simulink model "explicitCompFilter_uORB"  (R2024b)
settings: Solver=FixedStepAuto  StartTime=0.0  StopTime=35  FixedStep=0.005  RelTol=1e-3  EnableMultiTasking=on
PreLoadFcn:
  | %b_prev = Simulink.Signal;
  | %q_prev = Simulink.Signal;
  | 
  | %b_prev.InitialValue = '[0; 0; 0]';
  | %q_prev.InitialValue = '[0; 0; 0; 0]';
InitFcn:
  | %g_or = [0;0;-9.81];
  | %m_or = [27.5550; 2.4169; 16.0849];
  | gyroBias = [1; 1; 0.5];
  | 
  | %IF USING BUILT-IN UAV ANIMATION, uncomment below
  | 
  | %CLEAR UAV ANIMATIONS
  | %figHandles = findall(groot, 'Type', 'figure');
  | 
  | %for i=1:size(figHandles)
  | %    figObj = figHandles(i);
  | %    figName = figObj.Name;
  | %   if contains(figName, 'UAV Animation');
  | %        delete(figObj);
  | %    end
  | %end
undefined symbols (not defined in the file): g
libraries: robotcorelib x3, simulink_extras x3, px4Sensorslib x2, simulink x1, matrix_library x1, vrlib x1, px4uORBlib x1
(part 1 of 3)
settings Model: SimulationMode=external  ExtModeTrigDuration=10  Creator=Alyssa  LastModifiedBy=Alyssa
settings SolverCC: PositivePriorityOrder=on
settings OptimizationCC: BlockReduction=off  BooleanDataType=off  EnhancedBackFolding=on  PassReuseOutputArgsAs=Individual arguments  ZeroExternalMemoryAtStartup=off  ZeroInternalMemoryAtStartup=off  MaxStackSize=64  OptimizeBlockOrder=speed  DifferentSizesBufferReuse=on  OptimizationCustomize=off  EfficientTunableParamExpr=on
settings DebuggingCC: SaveWithParameterizedLinksMsg=none  UnderspecifiedInitializationDetection=Classic  MergeDetectMultiDrivingBlocksExec=none  SignalResolutionControl=TryResolveAllWithWarning  ParameterTunabilityLossMsg=error
settings HardwareCC: ProdBitPerPointer=32  ProdBitPerSizeT=32  ProdBitPerPtrDiffT=32  ProdLargestAtomicInteger=Long  ProdLargestAtomicFloat=Double  ProdWordSize=32  ProdLongLongMode=on  ProdHWDeviceType=ARM Compatible->ARM Cortex  TargetLargestAtomicInteger=Long  TargetLargestAtomicFloat=Double  TargetLongLongMode=on  TargetIntDivRoundTo=Zero  TargetEndianess=LittleEndian  TargetHWDeviceType=ARM Compatible->ARM Cortex
settings ModelReferenceCC: PropagateSignalLabelsOutOfModel=off
settings SFSimCC: MATLABDynamicMemAlloc=off  SimTargetLang=C++
settings RTWCC: Description=Embedded Coder  SystemTargetFile=ert.tlc  HardwareBoard=PX4 Pixhawk Series  TLCOptions="-aInlineSetEventsForThisBaseRateFcn=TLC_FALSE -aSuppressMultiTaskScheduler=TLC_FALSE  -aRateBasedStepFcn=0"  TemplateMakefile=ert_default_tmf  Toolchain=GNU Tools for PX4 Autopilots  TargetLang=C++
settings CodeAppCC: ForceParamTrailComments=on  IgnoreCustomStorageClasses=off  OperatorAnnotations=on  SimulinkDataObjDesc=on  SFDataObjDesc=on  InsertBlockDesc=on
settings ERTTargetCC: ExtModeTransport=3  ExtModeStaticAlloc=on  ExtModeStaticAllocSize=1024  ExtModeMexFile=ext_xcp  ExtModeIntrfLevel=Level2 - Open  InlinedParameterPlacement=Hierarchical  RootIOFormat=Structure reference

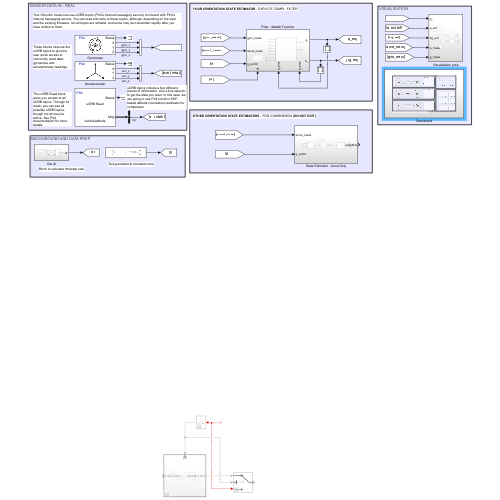
[thumbnail: Simulink's stored preview of the top-level diagram]
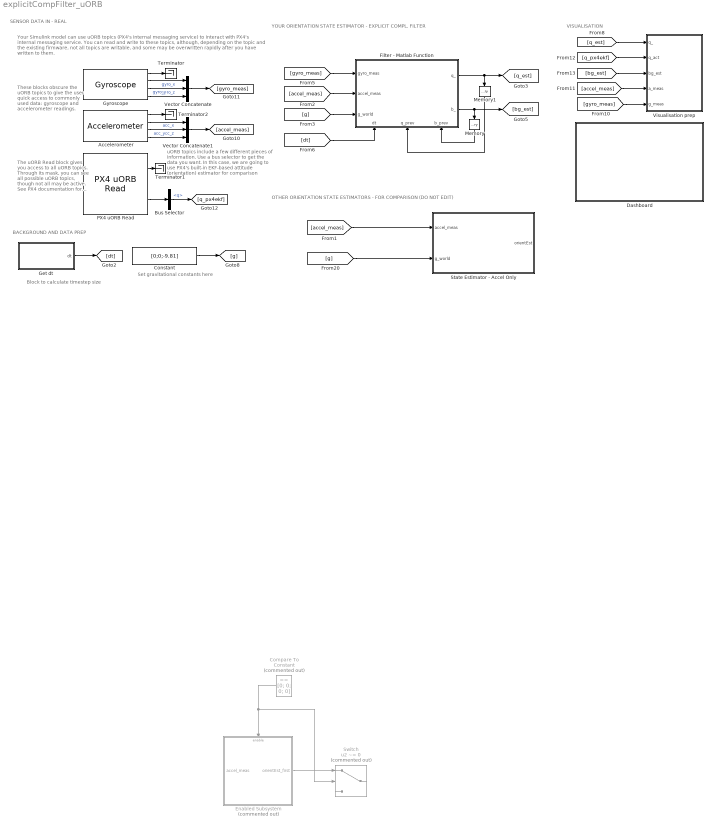
== system explicitCompFilter_uORB ==
  note: Set gravitational constants here
  note: Block to calculate timestep size
  note: uORB topics include a few different pieces of information. Use a bus selector to get the data you want. In this case, we are going to use PX4's built-in EKF-based attitude (orientation) estimator for comparison
  note: Your Simulink model can use uORB topics (PX4's internal messaging service) to interact with PX4's internal messaging service. You can read and write to these topics, although, depending on the topic and the existing firmware, not all topics are writable, and some may be overwritten rapidly after you have written to them.
  note: OTHER ORIENTATION STATE ESTIMATORS - FOR COMPARISON (DO NOT EDIT)
  note: VISUALISATION
  note: YOUR ORIENTATION STATE ESTIMATOR - EXPLICIT COMPL. FILTER
  note: BACKGROUND AND DATA PREP
  note: SENSOR DATA IN - REAL
  note: These blocks obscure the uORB topics to give the user quick access to commonly used data: gyroscope and accelerometer readings.
  note: The uORB Read block gives you access to all uORB topics. Through its mask, you can see all possible uORB topics, though not all may be active. See PX4 documentation for more details.
  Accelerometer : px4Sensorslib/Accelerometer  uorbTimeStamp=off  BlockingMode=off  BlockTimeout=1e-3  sampleTime=0.005
  Bus Selector : BusSelector  OutputSignals=q
  Compare To Constant : simulink/Logic and Bit Operations/Compare To Constant  Commented=on  relop===  const=[0; 0; 0; 0]  OutDataTypeStr=boolean
  Constant : Constant  Value=[0;0;-9.81]
  Dashboard : Subsystem
  Enabled Subsystem : Subsystem  Commented=on  TreatAsAtomicUnit=on
  Filter - Matlab Function : Subsystem
      settings: PortSchema="{\"entries\":[{\"content\":{\"sides\":[{\"content\":{\"connectorIds\":[\"In1\",\"In2\",\"In3\"]},\"type\":\"ConnectorPlacement.EquallySpacedRectSide\",\"uuid\":\"120bcc35-90e2-4731-ad16-59b67db11649\"},{\"content\":{\"connectorIds\":[\"Out1\",\"Out2\"],\"side\":\"RIGHT\"},\"type\":\"ConnectorPlacement.EquallySpacedRectSide\",\"uuid\":\"22d58821-716e-45cf-a51f-08f37bdaf288\"},{\"content\":{\"side\":\"TOP\"},\"type\":\"ConnectorPlacement.EquallySpacedRectSide\",\"uuid\":\"ed81b21f-3f84-420f-a2fc-1eb3e92691bd\"},{\"content\":{\"connectorIds\":[\"In4\",\"In5\",\"In6\"],\"side\":\"BOTTOM\"},\"type\":\"ConnectorPlacement.EquallySpacedRectSide\",\"uuid\":\"91ee1563-cd18-490d-aa8e-820150fc957e\"}]},\"type\":\"ConnectorPlacement.EquallySpacedConnector\",\"uuid\":\"c3e854d1-83c9-4500-85fa-dacad668fd3c\"}],\"packageUris\":[\"http://schema.mathworks.com/mf0/Connector/R2020b\"],\"version\":\"1.0\"}"
  Get dt : Subsystem
  Gyroscope : px4Sensorslib/Gyroscope  uorbTimeStamp=off  BlockingMode=off  BlockTimeout=1e-3  sampleTime=0.005
  Memory : Memory  InitialCondition=[0; 0; 0]
  Memory1 : Memory  InitialCondition=[1; 0; 0; 0]
  PX4 uORB Read : px4uORBlib/PX4 uORB Read  uORBTopic=VehicleAttitude  selectInstance=vehicle_attitude  SampleTime=-1  BlockingMode=off  BlockTimeout=1e-3
  State Estimator - Accel Only : Subsystem
  Switch : Switch  Commented=on  Criteria=u2 ~= 0  SaturateOnIntegerOverflow=off  InputSameDT=off
  Terminator : Terminator
  Terminator1 : Terminator
  Terminator2 : Terminator
  Vector Concatenate : Concatenate  NumInputs=3  Mode=Multidimensional array
  Vector Concatenate1 : Concatenate  NumInputs=3  Mode=Multidimensional array
  Visualisation prep : Subsystem
  wires:
  Enabled Subsystem/1(orientEst_first) -> Switch/1
  Compare To Constant/1 -> Enabled Subsystem/Enable, Switch/2
  ? -> Compare To Constant/1, Switch/3
  [accel_meas] -> State Estimator - Accel Only/1(accel_meas)
  [gyro_meas] -> Filter - Matlab Function/1(gyro_meas)
  [accel_meas] -> Filter - Matlab Function/2(accel_meas)
  Memory1/1 -> Filter - Matlab Function/5(q_prev)
  Memory/1 -> Filter - Matlab Function/6(b_prev)
  Filter - Matlab Function/2(b_) -> Memory/1, [bg_est]
  Filter - Matlab Function/1(q_) -> Memory1/1, [q_est]
  [dt] -> Filter - Matlab Function/4(dt)
  Gyroscope/2 -> Vector Concatenate/1  "gyro_x"
  Accelerometer/4 -> Vector Concatenate1/3  "acc_z"
  Gyroscope/4 -> Vector Concatenate/3  "gyro_z"
  Accelerometer/2 -> Vector Concatenate1/1  "acc_x"
  Gyroscope/3 -> Vector Concatenate/2  "gyro_y"
  Accelerometer/3 -> Vector Concatenate1/2  "acc_y"
  Vector Concatenate1/1 -> [accel_meas]
  PX4 uORB Read/2 -> Bus Selector/1
  Bus Selector/1 -> [q_px4ekf]  "<q>"
  Vector Concatenate/1 -> [gyro_meas]
  [q_px4ekf] -> Visualisation prep/2(q_act)
  [q_est] -> Visualisation prep/1(q_)
  [bg_est] -> Visualisation prep/3(bg_est)
  [accel_meas] -> Visualisation prep/4(a_meas)
  [gyro_meas] -> Visualisation prep/5(g_meas)
  Get dt/1(dt) -> [dt]
  Constant/1 -> [g]
  [g] -> Filter - Matlab Function/3(g_world)
  [g] -> State Estimator - Accel Only/2(g_world)
  Gyroscope/1 -> Terminator/1
  PX4 uORB Read/1 -> Terminator1/1
  Accelerometer/1 -> Terminator2/1
